simulink model "untitled7"  (Simulink 7.9)
settings: Solver=ode45  StartTime=0.0  StopTime=10.0  RelTol=1e-3
undefined symbols (not defined in the file or in its folder): D, j, Pilot_Level, QAM_Level
libraries: commrandsrc2 x1, dspxfrm3 x1, commdigbbndam3 x1
settings Model: Creator=Estilo  LastModifiedBy=Estilo

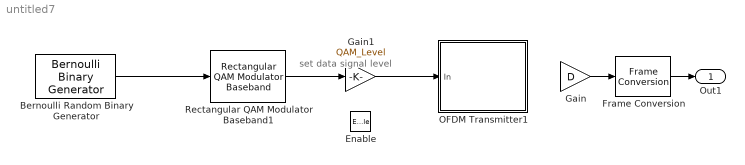
== system untitled7 ==
  note: set data signal level
  Enable : EnablePort
  Bernoulli Random Binary Generator : commrandsrc2/Bernoulli Binary Generator  P=0.5  seed=123  Ts=-1  frameBased=on  sampPerFrame=4  orient=off  outDataType=double
  Frame Conversion : FrameConversion  OutFrame=Sample-based
  Gain : Gain  Gain=D
  Gain1 : Gain  Gain=QAM_Level  SaturateOnIntegerOverflow=on  OutDataTypeStr=Inherit: Same as input  ParamDataTypeStr=Inherit: Same as input
  OFDM Transmitter1 : Subsystem
      mask Display: disp('OFDM\nTransmitter')
  Rectangular QAM Modulator Baseband1 : commdigbbndam3/Rectangular QAM Modulator Baseband  M=2  InType=Bit  Enc=Binary  Mapping=[0:15]  PowType=Min. distance between symbols  MinDist=2  AvgPow=1  PeakPow=1  Ph=0  outDtype=double  outWordLen=16  outUDDataType=sfix(16)  outFracLenMode=Best precision  outFracLen=15
  Out1 : Outport
  wires:
  Bernoulli Random Binary Generator/1 -> Rectangular QAM Modulator Baseband1/1
  Rectangular QAM Modulator Baseband1/1 -> Gain1/1
  Gain/1 -> Frame Conversion/1
  Frame Conversion/1 -> Out1/1
  Gain1/1 -> OFDM Transmitter1/1(In)

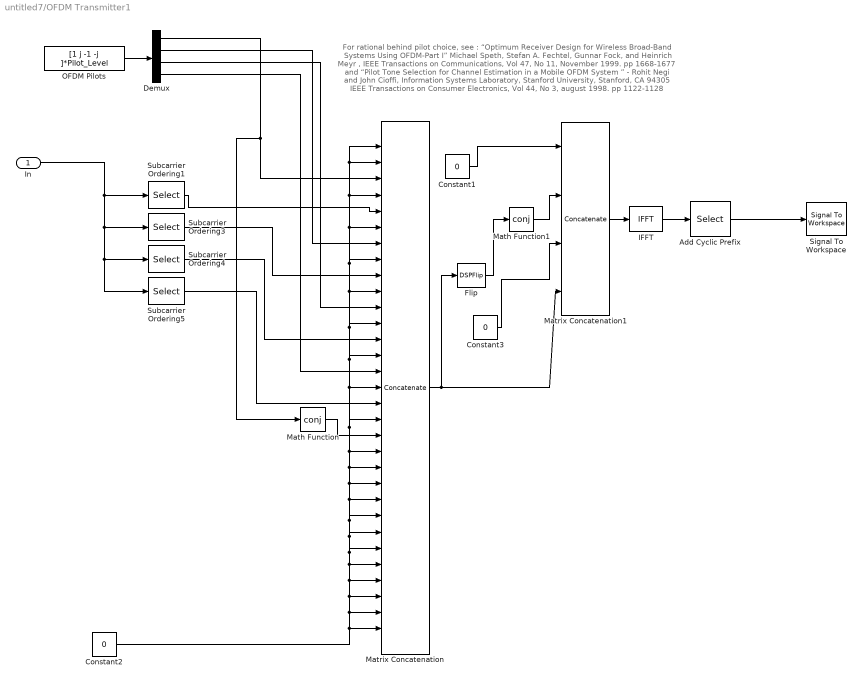
== system untitled7/OFDM Transmitter1 ==
  note: For rational behind pilot choice, see :
      | “Optimum Receiver Design for Wireless Broad-Band Systems Using OFDM-Part I”
      | Michael Speth, Stefan A. Fechtel, Gunnar Fock, and Heinrich Meyr ,
      |  IEEE Transactions on Communications, Vol 47, No 11, November 1999. pp 1668-1677
      | and
      | “Pilot Tone Selection for Channel Estimation in a Mobile OFDM System ” -
      |  Rohit Negi and John Cioffi, Information Systems Laboratory, Stanford University, Stanford, CA 94305
      | IEEE Transactions on Consumer Electronics, Vol 44, No 3, august 1998. pp 1122-1128
  In : Inport
  Add Cyclic Prefix : Selector  InputPortWidth=64  IndexOptions=Index vector (dialog)  Indices=[49:64 1:64]  OutputSizes=1
  Constant1 : Constant  Value=0
  Constant2 : Constant  Value=0
  Constant3 : Constant  Value=0
  Demux : Demux
  Flip : DSPFlip
  IFFT : dspxfrm3/IFFT  CompMethod=Table lookup  TableOpt=HYBRID  TableOptActive=Speed  BitRevOrder=off  cs_in=off  SkipNorm=on  InheritFFTLength=on  FFTLength=64  mode=Complex  outSamplingMode=Frame based  RowConvenienceOn=on  FFTImplementation=Auto  firstCoeffDataTypeStr=Inherit: Same word length as input  firstCoeffLastDataTypeStr=Inherit: Same word length as input  outputMin=[]  outputMax=[]  roundingMode=Floor  overflowMode=off
  Math Function : Math  Operator=conj  SaturateOnIntegerOverflow=on
  Math Function1 : Math  Operator=conj  SaturateOnIntegerOverflow=on
  Matrix Concatenation : Concatenate  NumInputs=31  Mode=Multidimensional array
  Matrix Concatenation1 : Concatenate  NumInputs=4  Mode=Multidimensional array
  OFDM Pilots : Constant  Value="[1 j -1 -j   ]*Pilot_Level"
  Signal To Workspace : SignalToWorkspace  VariableName=yout
      settings: CopyFcn=dspblkcopystw(gcbh);
  Subcarrier Ordering1 : Selector  InputPortWidth=4  IndexOptions=Index vector (dialog)  Indices=1  OutputSizes=1
  Subcarrier Ordering3 : Selector  InputPortWidth=4  IndexOptions=Index vector (dialog)  Indices=2  OutputSizes=1
  Subcarrier Ordering4 : Selector  InputPortWidth=4  IndexOptions=Index vector (dialog)  Indices=3  OutputSizes=1
  Subcarrier Ordering5 : Selector  InputPortWidth=4  IndexOptions=Index vector (dialog)  Indices=4  OutputSizes=1
  wires:
  In/1 -> Subcarrier Ordering4/1, Subcarrier Ordering5/1, Subcarrier Ordering3/1, Subcarrier Ordering1/1
  IFFT/1 -> Add Cyclic Prefix/1
  Add Cyclic Prefix/1 -> Signal To Workspace/1
  OFDM Pilots/1 -> Demux/1
  Demux/1 -> Matrix Concatenation/3, Math Function/1
  Subcarrier Ordering1/1 -> Matrix Concatenation/5
  Demux/2 -> Matrix Concatenation/7
  Subcarrier Ordering3/1 -> Matrix Concatenation/9
  Demux/3 -> Matrix Concatenation/11
  Subcarrier Ordering4/1 -> Matrix Concatenation/13
  Demux/4 -> Matrix Concatenation/15
  Subcarrier Ordering5/1 -> Matrix Concatenation/17
  Constant2/1 -> Matrix Concatenation/31, Matrix Concatenation/30, Matrix Concatenation/29, Matrix Concatenation/28, Matrix Concatenation/27, Matrix Concatenation/26, Matrix Concatenation/25, Matrix Concatenation/24, Matrix Concatenation/23, Matrix Concatenation/22, Matrix Concatenation/21, Matrix Concatenation/20, Matrix Concatenation/18, Matrix Concatenation/16, Matrix Concatenation/14, Matrix Concatenation/12, Matrix Concatenation/10, Matrix Concatenation/8, Matrix Concatenation/6, Matrix Concatenation/4, Matrix Concatenation/1, Matrix Concatenation/2
  Math Function/1 -> Matrix Concatenation/19
  Constant1/1 -> Matrix Concatenation1/1
  Matrix Concatenation/1 -> Flip/1, Matrix Concatenation1/4
  Flip/1 -> Math Function1/1
  Math Function1/1 -> Matrix Concatenation1/2
  Constant3/1 -> Matrix Concatenation1/3
  Matrix Concatenation1/1 -> IFFT/1
